simulink model "LAB2_1"  (R2020b)
settings: Solver=FixedStepDiscrete  StartTime=0.0  StopTime=30  FixedStep=0.0001  RelTol=1e-3
values from neighbouring files (symbols this model uses):
  Kd = place(Ad, Bd, polesK_d)    [DiscreteSS.m]    (also in PIDparam.m = Kp*Td)
  Ki = Kp/Ti    [PIDparam.m]
  Kp = delta_K*cos(delta_phi)    [PIDparam.m]
  Kw = 1/Tw    [PIDparam.m]
  Ts = 0.001    [DiscreteSS.m]    (also in discretePID.m; regulatorDT.m = 0.05)
undefined symbols (not defined in the file or in its folder): BeqEst, denC_d, DiscIntNeverNeededParam, drv, gbox, JeqEst, mot, National_Instruments, numC_d, PCI, Req, rpm2degs, rpm2rads, sens, tauSfEst, Tl
libraries: sldrtlib x3, simulink x1
settings Model: ExtModeTrigDuration=10001  Creator=umbe  LastModifiedBy=giorgiadisaro
settings HardwareCC: ProdBitPerLong=64  ProdHWDeviceType=Intel->x86-64 (Mac OS X)
settings RTWCC: Description=Simulink Desktop Real-Time  SystemTargetFile=sldrt.tlc  TemplateMakefile=sldrt.tmf  RTWCompilerOptimization=on
settings CodeAppCC: MaxIdLength=95
settings SimulinkDesktopRealTimeCC: TargetPreCompLibLocation=/Applications/MATLAB_R2020b.app/toolbox/sldrt/lib/maci64

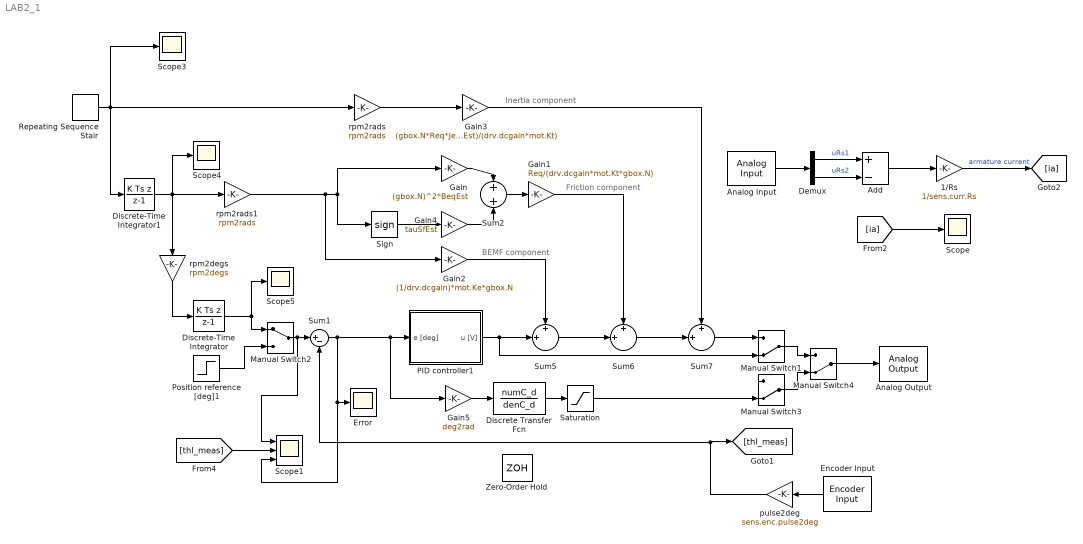
== system LAB2_1 ==
  note: Inertia component
  note: Friction component
  note: BEMF component
  1/Rs : Gain  Gain=1/sens.curr.Rs
  Add : Sum  Inputs=+-
  Analog Input : sldrtlib/Analog Input  SampleTime=-1  MaxMissedTicks=10  ShowMissedTicks=off  YieldWhenWaiting=off  DrvName=National_Instruments/PCI-6221  DrvAddress=4294967295  DrvOptions=[0 0 0 2 0]  Channels=[1 2]  RangeMode=1  VoltRange=1  DataType=1
      settings: AttributesFormatString=National Instruments\nPCI-6221 [auto]
  Analog Output : sldrtlib/Analog Output  SampleTime=-1  MaxMissedTicks=10  ShowMissedTicks=off  YieldWhenWaiting=off  DrvName=National_Instruments/PCI-6221  DrvAddress=4294967295  DrvOptions=[0 0 0 2 0]  Channels=1  RangeMode=1  VoltRange=1  InitialValue=0  FinalValue=0
      settings: AttributesFormatString=National Instruments\nPCI-6221 [auto]
  Demux : Demux  Outputs=2
  Discrete Transfer Fcn : DiscreteTransferFcn  Numerator=numC_d  Denominator=denC_d  SampleTime=Ts
  Discrete-Time Integrator : DiscreteIntegrator  IntegratorMethod=Integration: Backward Euler  SampleTime=Ts  ICPrevOutput=DiscIntNeverNeededParam  ICPrevScaledInput=DiscIntNeverNeededParam
  Discrete-Time Integrator1 : DiscreteIntegrator  IntegratorMethod=Integration: Backward Euler  SampleTime=Ts  ICPrevOutput=DiscIntNeverNeededParam  ICPrevScaledInput=DiscIntNeverNeededParam
  Encoder Input : sldrtlib/Encoder Input  SampleTime=-1  MaxMissedTicks=10  ShowMissedTicks=off  YieldWhenWaiting=off  DrvName=National_Instruments/PCI-6221  DrvAddress=4294967295  DrvOptions=[0 0 0 2 0]  Channels=1  QuadMode=3  IndexPulse=1  InputFilter=Inf  DataType=1
      settings: AttributesFormatString=National Instruments\nPCI-6221 [auto]
  Error : Scope
  Gain : Gain  Gain=(gbox.N)^2*BeqEst
  Gain1 : Gain  Gain=Req/(drv.dcgain*mot.Kt*gbox.N)
  Gain2 : Gain  Gain=(1/drv.dcgain)*mot.Ke*gbox.N
  Gain3 : Gain  Gain=(gbox.N*Req*JeqEst)/(drv.dcgain*mot.Kt)
  Gain4 : Gain  Gain=tauSfEst
  Gain5 : Gain  Gain=deg2rad
  Manual Switch1 : ManualSwitch  CurrentSetting=0
  Manual Switch2 : ManualSwitch
  Manual Switch3 : ManualSwitch  CurrentSetting=0
  Manual Switch4 : ManualSwitch  CurrentSetting=0
  PID controller1 : Subsystem
  Position reference [deg]1 : Step  After=360  SampleTime=Ts
  Repeating Sequence Stair : simulink/Sources/Repeating Sequence Stair  OutValues=[900 0 -900 -900 0 900].'  tsamp=0.5  OutMin=[]  OutMax=[]  OutDataTypeStr=double  OutputDataTypeScalingMode=double  OutDataType=fixdt(0,8)  ConRadixGroup=Best Precision: Vector-wise  OutScaling=2^-12
  Saturation : Saturate  UpperLimit=10  LowerLimit=-10
  Scope{,3..5} (4 alike) : Scope
  Scope1 : Scope  NumInputPorts=3
  Sign : Signum
  Sum1 : Sum  Inputs=|+-
  Sum2 : Sum  Inputs=+|+
  Sum5 : Sum  Inputs=+|+||
  Sum6 : Sum  Inputs=+|+||
  Sum7 : Sum  Inputs=+|+||
  Zero-Order Hold : ZeroOrderHold  SampleTime=Ts
  pulse2deg : Gain  Gain=sens.enc.pulse2deg
  rpm2degs : Gain  Gain=rpm2degs
  rpm2rads : Gain  Gain=rpm2rads
  rpm2rads1 : Gain  Gain=rpm2rads
  wires:
  1/Rs/1 -> [ia]  "armature current"
  Add/1 -> 1/Rs/1
  Demux/1 -> Add/1  "uRs1"
  Demux/2 -> Add/2  "uRs2"
  pulse2deg/1 -> Sum1/2, [thl_meas]
  [ia] -> Scope/1
  Encoder Input/1 -> pulse2deg/1
  Analog Input/1 -> Demux/1
  Gain1/1 -> Sum6/1
  Gain4/1 -> Sum2/2
  Manual Switch2/1 -> Scope1/1, Sum1/1
  Sum1/1 -> Scope1/3, Error/1, Gain5/1, PID controller1/1(e [deg])
  rpm2degs/1 -> Discrete-Time Integrator/1
  Sum2/1 -> Gain1/1
  Repeating Sequence Stair/1 -> Scope3/1, Discrete-Time Integrator1/1, rpm2rads/1
  Gain3/1 -> Sum7/1
  Gain/1 -> Sum2/1
  rpm2rads1/1 -> Gain2/1, Sign/1, Gain/1
  Position reference [deg]1/1 -> Manual Switch2/2
  Sum7/1 -> Manual Switch1/1
  Discrete-Time Integrator1/1 -> Scope4/1, rpm2rads1/1, rpm2degs/1
  rpm2rads/1 -> Gain3/1
  Discrete-Time Integrator/1 -> Scope5/1, Manual Switch2/1
  PID controller1/1(u [V]) -> Manual Switch1/2, Sum5/2
  Gain2/1 -> Sum5/1
  Sign/1 -> Gain4/1
  Sum5/1 -> Sum6/2
  Sum6/1 -> Sum7/2
  Gain5/1 -> Discrete Transfer Fcn/1
  Discrete Transfer Fcn/1 -> Saturation/1
  Saturation/1 -> Manual Switch3/2
  Manual Switch1/1 -> Manual Switch4/1
  Manual Switch3/1 -> Manual Switch4/2
  Manual Switch4/1 -> Analog Output/1
  [thl_meas] -> Scope1/2

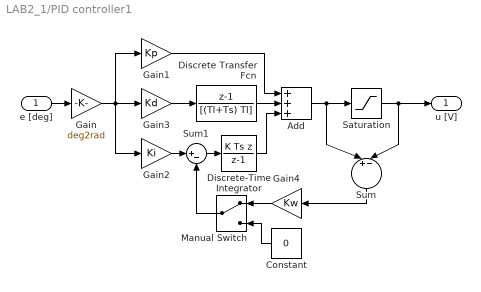
== system LAB2_1/PID controller1 ==
  e [deg] : Inport
  Add : Sum  Inputs=+++
  Constant : Constant  Value=0
  Discrete Transfer Fcn : DiscreteTransferFcn  Numerator=[1 -1]  Denominator=[(Tl+Ts) Tl]  SampleTime=Ts
  Discrete-Time Integrator : DiscreteIntegrator  IntegratorMethod=Integration: Backward Euler  SampleTime=Ts  ICPrevOutput=DiscIntNeverNeededParam  ICPrevScaledInput=DiscIntNeverNeededParam
  Gain : Gain  Gain=deg2rad
  Gain1 : Gain  Gain=Kp
  Gain2 : Gain  Gain=Ki
  Gain3 : Gain  Gain=Kd
  Gain4 : Gain  Gain=Kw
  Manual Switch : ManualSwitch
  Saturation : Saturate  UpperLimit=10  LowerLimit=-10
  Sum : Sum  Inputs=||+-||
  Sum1 : Sum  Inputs=|+-
  u [V] : Outport
  wires:
  Gain/1 -> Gain3/1, Gain1/1, Gain2/1
  Gain1/1 -> Add/1
  e [deg]/1 -> Gain/1
  Add/1 -> Sum/1, Saturation/1
  Saturation/1 -> Sum/2, u [V]/1
  Gain3/1 -> Discrete Transfer Fcn/1
  Sum1/1 -> Discrete-Time Integrator/1
  Gain2/1 -> Sum1/1
  Sum/1 -> Gain4/1
  Gain4/1 -> Manual Switch/1
  Manual Switch/1 -> Sum1/2
  Constant/1 -> Manual Switch/2
  Discrete-Time Integrator/1 -> Add/3
  Discrete Transfer Fcn/1 -> Add/2
